simulink model "ECSE308_Lab_2_1_1"  (R2019b)
settings: Solver=VariableStepAuto  StartTime=0.0  StopTime=10.0  RelTol=1e-3
libraries: commchan3 x1, dsparch4 x1
settings Model: Creator=mikewang  LastModifiedBy=mikewang

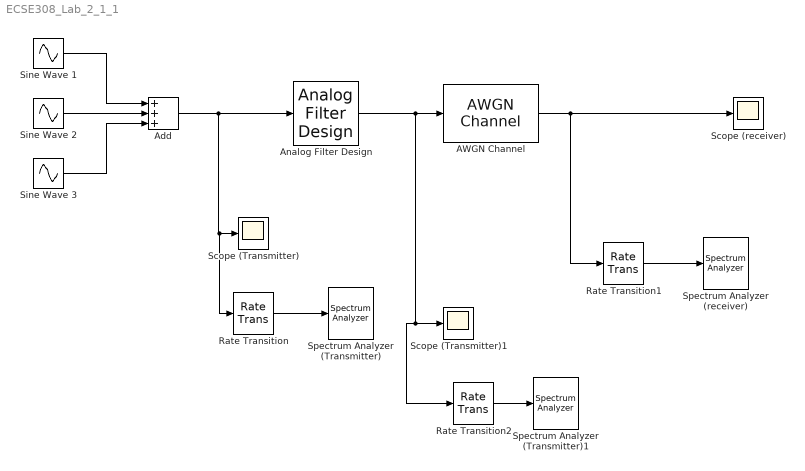
== system ECSE308_Lab_2_1_1 ==
  AWGN Channel : commchan3/AWGN Channel  InputProcessing=Columns as channels (frame based)  seed=randseed  noiseMode=Variance from mask  EbNodB=10  EsNodB=10  SNRdB=10  bitsPerSym=1  Ps=1  Tsym=1  variance=1e-3
      settings: SourceProductName=Communications Toolbox
  "Add " : Sum  Inputs=+++
  "Analog Filter Design " : dsparch4/Analog Filter Design  method=Butterworth  filttype=Bandpass  N=8  Wlo=pi  Whi=1000*pi  Rp=2  Rs=40
  Rate Transition : RateTransition  OutPortSampleTime=1/50000
  Rate Transition1 : RateTransition  OutPortSampleTime=1/50000
  Rate Transition2 : RateTransition  OutPortSampleTime=1/50000
  Scope (Transmitter) : Scope
  Scope (Transmitter)1 : Scope
  Scope (receiver) : Scope
  Sine Wave 1 : Sin  Amplitude=0.5  Frequency=1000*pi  SampleTime=0
  Sine Wave 2 : Sin  Amplitude=0.2  Frequency=600*pi  SampleTime=0
  Sine Wave 3 : Sin  Amplitude=0.3  Frequency=1200*pi  SampleTime=0
  Spectrum Analyzer (Transmitter) : SpectrumAnalyzer
  Spectrum Analyzer (Transmitter)1 : SpectrumAnalyzer
  Spectrum Analyzer (receiver) : SpectrumAnalyzer
  wires:
  Sine Wave 1/1 -> "Add "/1
  Sine Wave 2/1 -> "Add "/2
  Sine Wave 3/1 -> "Add "/3
  "Add "/1 -> Rate Transition/1, Scope (Transmitter)/1, "Analog Filter Design "/1
  Rate Transition/1 -> Spectrum Analyzer (Transmitter)/1
  AWGN Channel/1 -> Rate Transition1/1, Scope (receiver)/1
  Rate Transition1/1 -> Spectrum Analyzer (receiver)/1
  Rate Transition2/1 -> Spectrum Analyzer (Transmitter)1/1
  "Analog Filter Design "/1 -> Scope (Transmitter)1/1, Rate Transition2/1, AWGN Channel/1
